simulink model "TrayectoriaPurePursuitM"  (R2023b)
settings: Solver=FixedStepAuto  StartTime=0.0  StopTime=150  RelTol=1e-3  EnableMultiTasking=on
model workspace (MAT data in the model file):
  d = 0.189
libraries: slpidlib x1
settings Model: PacingRate=5  ExtModeTrigDuration=2  Creator=juana  LastModifiedBy=juana
settings OptimizationCC: EnhancedBackFolding=on  PassReuseOutputArgsAs=Individual arguments  ZeroExternalMemoryAtStartup=off  ZeroInternalMemoryAtStartup=off  MaxStackSize=64  OptimizeBlockOrder=speed  DifferentSizesBufferReuse=on  EfficientTunableParamExpr=on
settings DebuggingCC: ParameterTunabilityLossMsg=error
settings HardwareCC: ProdBitPerInt=16  ProdBitPerPointer=16  ProdBitPerSizeT=16  ProdBitPerPtrDiffT=16  ProdLargestAtomicFloat=None  ProdWordSize=8  ProdHWDeviceType=Atmel->AVR  UseEmbeddedCoderFeatures=off  UseSimulinkCoderFeatures=off
settings SFSimCC: MATLABDynamicMemAlloc=off
settings RTWCC: Description=Embedded Coder  SystemTargetFile=ert.tlc  HardwareBoard=Arduino Mega 2560  TemplateMakefile=ert_default_tmf  Toolchain=Arduino AVR  BuildConfiguration=Faster Runs
settings CodeAppCC: ForceParamTrailComments=on  IgnoreCustomStorageClasses=off  OperatorAnnotations=on  SimulinkDataObjDesc=on  SFDataObjDesc=on  MangleLength=10  InsertBlockDesc=on
settings ERTTargetCC: SupportContinuousTime=on  SupportNonInlinedSFcns=on  SupportVariableSizeSignals=on  ExtModeTransport=3  ExtModeStaticAlloc=on  ExtModeAutomaticAllocSize=off  ExtModeStaticAllocSize=2048  ExtModeMexFile=ext_xcp  ExtModeIntrfLevel=Level2 - Open

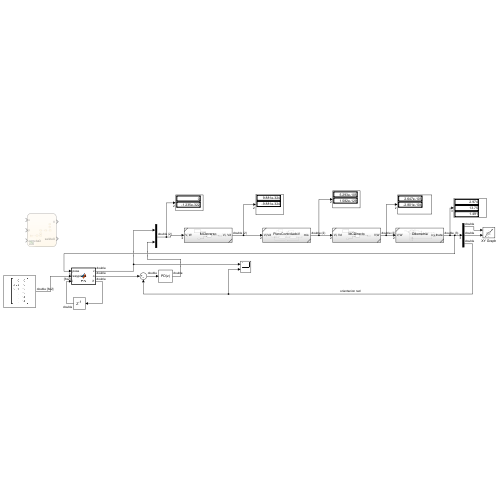
[thumbnail: Simulink's stored preview of the top-level diagram]
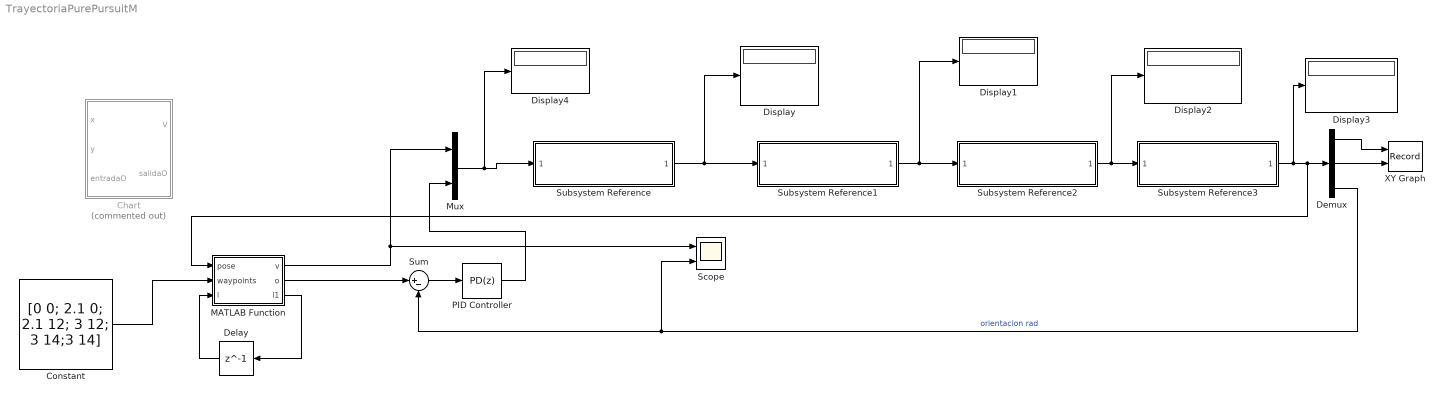
== system TrayectoriaPurePursuitM ==
  Chart : Stateflow chart  Commented=on  TreatAsAtomicUnit=on
      settings: PortSchema="{\"entries\":[{\"content\":{\"sides\":[{\"content\":{\"connectorIds\":[\"In1\",\"In3\",\"In2\"]},\"type\":\"ConnectorPlacement.EquallySpacedRectSide\",\"uuid\":\"97edc7af-c120-4b1b-8699-fb281b336c5f\"},{\"content\":{\"connectorIds\":[\"Out1\",\"Out2\"],\"side\":\"RIGHT\"},\"type\":\"ConnectorPlacement.EquallySpacedRectSide\",\"uuid\":\"66ab9f46-ef7c-4995-b93c-2ccdd63331e6\"},{\"content\":{\"side\":\"TOP\"},\"type\":\"ConnectorPlacement.EquallySpacedRectSide\",\"uuid\":\"7d6396ab-5886-4c89-b447-2228444dcfb9\"}]},\"type\":\"ConnectorPlacement.EquallySpacedConnector\",\"uuid\":\"f9e2802f-7001-4f64-94f0-930e28ba0fbf\"}],\"packageUris\":[\"http://schema.mathworks.com/mf0/Connector/R2020b\"],\"version\":\"1.0\"}"
  Constant : Constant  Value=[0 0; 2.1 0; 2.1 12; 3 12; 3 14;3 14]
  Delay : Delay  DelayLength=1
  Demux : Demux  Outputs=3
  Display{,1..4} (5 alike) : Display
  MATLAB Function : MATLAB Function  TreatAsAtomicUnit=on
  Mux : Mux  Inputs=2
  PID Controller : slpidlib/PID Controller  Controller=PD  Form=Parallel  TimeDomain=Discrete-time  UseExternalTs=off  SampleTime=-1  IntegratorMethod=Forward Euler  FilterMethod=Forward Euler  ControllerParametersSource=internal  P=2.93953075898814  I=0.639832143442781  UseKiTs=off  D=0.80184050447165  N=24.9099900076981  UseFilter=on  TunerSelectOption=Transfer Function Based (PID Tuner App)  InitialConditionSource=internal  InitialConditionForIntegrator=0  InitialConditionForFilter=0  DifferentiatorICPrevScaledInput=0  ExternalReset=none  TrackingMode=off  Kt=1  LimitOutput=off  SatLimitsSource=internal  UpperSaturationLimit=inf  LowerSaturationLimit=-inf  LinearizeAsGain=on  AntiWindupMode=none  Kb=1  LimitIntegrator=off  UpperIntegratorSaturationLimit=inf  LowerIntegratorSaturationLimit=-inf  POutMin=[]  POutMax=[]  IOutMin=[]  IOutMax=[]  DOutMin=[]  DOutMax=[]  NOutMin=[]  NOutMax=[]  SumOutMin=[]  SumOutMax=[]  SaturationOutMin=[]  SaturationOutMax=[]  PParamMin=[]  PParamMax=[]  IParamMin=[]  IParamMax=[]  DParamMin=[]  DParamMax=[]  NParamMin=[]  NParamMax=[]  KbParamMin=[]  KbParamMax=[]  KtParamMin=[]  KtParamMax=[]  KbOutMin=[]  KbOutMax=[]  KtOutMin=[]  KtOutMax=[]  IntegratorOutMin=[]  IntegratorOutMax=[]  FilterOutMin=[]  FilterOutMax=[]  SumI1OutMin=[]  SumI1OutMax=[]  SumI2OutMin=[]  SumI2OutMax=[]  SumI3OutMin=[]  SumI3OutMax=[]  SumI4OutMin=[]  SumI4OutMax=[]  SumDOutMin=[]  SumDOutMax=[]  DifferentiatorOutMin=[]  DifferentiatorOutMax=[]  FilterDiffOutCoefMin=[]  FilterDiffOutCoefMax=[]  ReciprocalOutMin=[]  ReciprocalOutMax=[]  SumDenOutMin=[]  SumDenOutMax=[]  SumNumOutMin=[]  SumNumOutMax=[]  DivideOutMin=[]  DivideOutMax=[]  UdiffTsProdOutMin=[]  UdiffTsProdOutMax=[]  NTsProdOutMin=[]  NTsProdOutMax=[]  UintegralTsProdOutMin=[]  UintegralTsProdOutMax=[]  UngainTsProdOutMin=[]  UngainTsProdOutMax=[]  ClampingZeroOutDataTypeStr=Inherit: Inherit via back propagation  ClampingZeroOutMin=[]  ClampingZeroOutMax=[]  FilterDenConstantOutDataTypeStr=Inherit: Inherit via back propagation  FilterDenConstantOutMin=[]  FilterDenConstantOutMax=[]  PCopyOutDataTypeStr=Inherit: Inherit via back propagation  PCopyOutMin=[]  PCopyOutMax=[]  NCopyOutDataTypeStr=Inherit: Inherit via back propagation  NCopyOutMin=[]  NCopyOutMax=[]  IntegratorContinuousStateAttributes=''  IntegratorStateMustResolveToSignalObject=off  IntegratorRTWStateStorageClass=Auto  FilterContinuousStateAttributes=''  FilterStateMustResolveToSignalObject=off  FilterRTWStateStorageClass=Auto  ParallelPVariant=InternalParameters  IdealPVariant=Disabled  IVariant=Disabled  DVariant=InternalParameters  IntegratorVariant=Disabled  SatVariant=Disabled  AWVariant=Disabled  PCopyVariant=Disabled  TRVariant=Disabled  FdbkBlocksVariant=Forward  IdealPFdbkVariant=Disabled  SatFdbkVariant=Disabled  DerivativeFilterVariant=ForwardEulerFilter  NVariant=InternalParameters  NCopyVariant=Disabled  FilterICVariant=InternalICsFilter  IntegratorICVariant=Disabled  ExternalResetVariant=Disabled  TRSumVariant=Passthrough  SumFdbkVariant=Disabled  SumVariant=Sum_PD  TsampFilterVariant=InternalTs  TsampNgainVariant=Passthrough  TsampIntegralVariant=Disabled_SignalSpec  ExternalSaturationOutDataTypeStr=Inherit: Same as second input
  Scope : Scope  NumInputPorts=2
  Subsystem Reference : Subsystem  ReferencedSubsystem=MCInverso
  Subsystem Reference1 : Subsystem  ReferencedSubsystem=PieroControladoV
  Subsystem Reference2 : Subsystem  ReferencedSubsystem=MCDirecto
  Subsystem Reference3 : Subsystem  ReferencedSubsystem=Odometria
  Sum : Sum  Inputs=|+-
  XY Graph : Record  FileSettingsInternal="{\"entries\":[{\"content\":{\"excelSettings\":{\"content\":{},\"type\":\"Streamout.ExcelSettings\"}},\"type\":\"Streamout.FileSettingStorage\",\"uuid\":\"\"}],\"packageUris\":[\"http:\\/\\/schema.mathworks.com\\/mf0\\/streamout_blocks\\/R2020a\"],\"version\":\"1.0\"}"  Layout=[1 1]  SignalsInternal="{\"entries\":[{\"content\":{\"signals\":[{\"content\":{\"blockPath\":[],\"dimensions\":[1],\"domain\":\"\",\"lineColor\":\"#a2142f\",\"plots\":[ 1 ],\"port\":1,\"signalID\":1,\"signalName\":\"Demux:1\"},\"type\":\"RecordBlkView.Signal\",\"uuid\":\"\"},{\"content\":{\"blockPath\":[],\"dimensions\":[1],\"domain\":\"\",\"lineColor\":\"#139fff\",\"plots\":[ 1 ],\"port\":2,\"signalID\":2,\"signalName\":\"Demux:2\"},\"type\":\"RecordBlkView.Signal\",\"uuid\":\"\"}]},\"type\":\"RecordBlkView.InputSignals\",\"uuid\":\"\"}],\"packageUris\":[\"http:\\/\\/schema.mathworks.com\\/mf0\\/streamout_blocks\\/R2020a\"],\"version\":\"1.0\"}"  VisualizationBindings="{\"xyplotplugin\":{\"info\":[{\"series\":[{\"bindingParametersList\":[{\"parameter\":\"X-Axis\",\"signalID\":1,\"signalName\":\"Demux:1\"},{\"parameter\":\"Y-Axis\",\"signalID\":2,\"signalName\":\"Demux:2\"}],\"seriesID\":0}],\"subplotID\":1}]}}"  CompatibilityTag=XY
  wires:
  Subsystem Reference1/1 -> Display1/1, Subsystem Reference2/1
  Subsystem Reference2/1 -> Display2/1, Subsystem Reference3/1
  Subsystem Reference/1 -> Display/1, Subsystem Reference1/1
  Subsystem Reference3/1 -> Display3/1, MATLAB Function/1(pose), Demux/1
  Demux/1 -> XY Graph/1
  Demux/2 -> XY Graph/2
  Demux/3 -> Scope/2, Sum/2  "orientacion rad"
  Mux/1 -> Display4/1, Subsystem Reference/1
  Sum/1 -> PID Controller/1
  MATLAB Function/1(v) -> Mux/1, Scope/1
  Constant/1 -> MATLAB Function/2(waypoints)
  PID Controller/1 -> Mux/2
  MATLAB Function/2(o) -> Sum/1
  Delay/1 -> MATLAB Function/3(i)
  MATLAB Function/3(i1) -> Delay/1

== matlab function TrayectoriaPurePursuitM/MATLAB Function ==
  data: v output double size=1; o output size=1; i1 output size=1; pose input; waypoints input; i input size=1
function [v, o, i1] = fcn(pose, waypoints, i)
%#codegen
LA=0.30;
%if isempty (indice) 
   % persistent indice = 0;
v = 0.205;
i = i+1;
i1=0;
x = pose(1);
y = pose(2);
O = pose(3);

if(length(waypoints) >= i)
    distancia=sqrt((waypoints(i,1)-x)^2 + (waypoints(i,2)-y)^2);
    while(distancia < LA) && (length(waypoints)>i)
        i=i+1;
        distancia = sqrt((waypoints(i,1)-x)^2 + (waypoints(i,2)-y)^2);
        v = 0.1;
    end
    o=atan2(waypoints(i,2)-y, waypoints(i,1)-x);
else
    o=pose(3);
    v=0;
end
if(length(waypoints) > i)
    i1=i-1;
else
    i1=i;
end

== stateflow chart TrayectoriaPurePursuitM/Chart ==
  state Paro
    salidaO=pi/2;
    V=0;
  state recto4
    V=0.205;
    salidaO=pi/2;
  state GiroDcha
    V = 0.10;
    salidaO=0;
  state recto1
    V=0.205;
    salidaO=0;
  state GiroIzq1
    V=0.205;
    salidaO=pi/2;
  state recto12
    V=0.205;
    salidaO=pi/2;
  state Marcha
    entry:
    V = 0.205;
    salidaO = 0;
  state GiroIzq
    V = 0.10;
    salidaO = pi/2;
  state Inicio
    V = 0;
    salidaO = 0;
  recto4 -> Paro : [y>14]
  GiroIzq1 -> recto4 : [entradaO>pi/2.00001]
  recto1 -> GiroIzq1 : [x>3]
  GiroDcha -> recto1 : [entradaO>0]
  recto12 -> GiroDcha : [y>12]
  GiroIzq -> recto12 : [entradaO>pi/2.0001]
  (default) -> Inicio
  Marcha -> GiroIzq : [x>1.7]
  Inicio -> Marcha : [after(1, sec)]
  data: V output double size=1 =0; salidaO output double size=1 =0; x input double size=1; entradaO input double size=1; y input double size=1
